simulink subsystem "phi_r_observer_current"  (R2022b)
settings: Solver=VariableStepAuto  StartTime=0.0  StopTime=10.0  RelTol=1e-3
undefined symbols (not defined in the file or in its folder): K5, K6
settings Model: Creator=jack  LastModifiedBy=jack

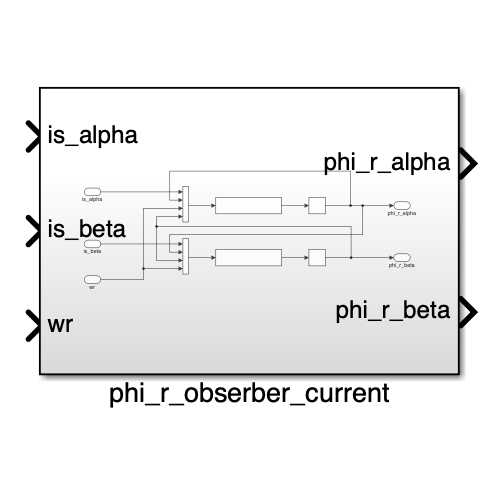
[thumbnail: Simulink's stored preview of the top-level diagram]
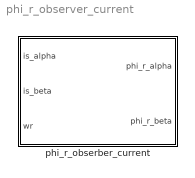
== system phi_r_observer_current ==
  phi_r_obserber_current : Subsystem

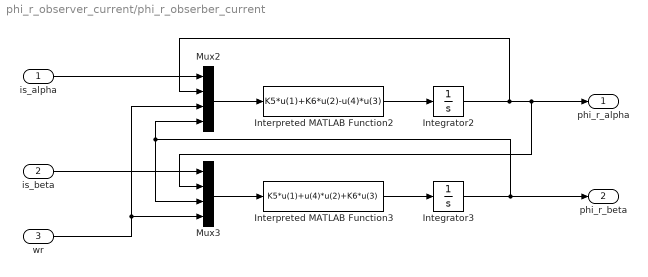
== system phi_r_observer_current/phi_r_obserber_current ==
  is_alpha : Inport
  is_beta : Inport  Port=2
  wr : Inport  Port=3
  Integrator2 : Integrator
  Integrator3 : Integrator
  Interpreted MATLAB Function2 : MATLABFcn  MATLABFcn=K5*u(1)+K6*u(2)-u(4)*u(3)
  Interpreted MATLAB Function3 : MATLABFcn  MATLABFcn=K5*u(1)+u(4)*u(2)+K6*u(3)
  Mux2 : Mux
  Mux3 : Mux
  phi_r_alpha : Outport
  phi_r_beta : Outport  Port=2
  wires:
  is_beta/1 -> Mux3/1
  wr/1 -> Mux3/4, Mux2/3
  is_alpha/1 -> Mux2/1
  Mux2/1 -> Interpreted MATLAB Function2/1
  Integrator3/1 -> phi_r_beta/1, Mux3/3, Mux2/4
  Integrator2/1 -> Mux2/2, phi_r_alpha/1, Mux3/2
  Interpreted MATLAB Function2/1 -> Integrator2/1
  Mux3/1 -> Interpreted MATLAB Function3/1
  Interpreted MATLAB Function3/1 -> Integrator3/1
